simulink model "hcu_main_ADASwEPS"  (Simulink 8.2)
settings: Solver=FixedStepDiscrete  StartTime=0.0  StopTime=inf  FixedStep=0.001  RelTol=1e-3
PostLoadFcn:
  | , if any(exist('dsrtsu_mdlpostloadfcn', 'file') == [2, 3, 6]), try dsrtsu_mdlpostloadfcn('Execute', bdroot); catch fprintf('Error in PostLoadFcn (dsrtsu_mdlpostloadfcn) for model "%s":\n %s\n', bdroot, lasterr); end, end,
values from neighbouring files (symbols this model uses):
  C_TASK_1MS_S = (	C_TICK_TIME_S       )    [hcu_local_hdr.m]    (also in temp_ovrd_values.m = double(	0.001                  ))
  C_TASK_5MS_S = (	C_TICK_TIME_S      	)    [hcu_local_hdr.m]
  ENUM_ADASLFCSTATUS_OFF = uint8(  0  )    [hcu_local_hdr.m]
  ENUM_ADASLFCSTATUS_STANDBY = uint8(  1  )    [hcu_local_hdr.m]
  ENUM_ADASLKASTATUS_ACTIVE = uint8(  2  )    [hcu_local_hdr.m]
  ENUM_ADASLKASTATUS_OFF = uint8(  0  )    [hcu_local_hdr.m]
  ENUM_ADASLKASTATUS_STANDBY = uint8(  1  )    [hcu_local_hdr.m]
  ENUM_EPSMODEREQ_ANGLE = uint8(  1  )    [hcu_local_hdr.m]
  ENUM_EPSMODEREQ_INTERNAL = uint8(  0  )    [hcu_local_hdr.m]
  ENUM_EPSMODEREQ_TORQUE = uint8(  2  )    [hcu_local_hdr.m]
  ENUM_GEARPOSN_1ST = uint8(  1  )    [hcu_local_hdr.m]
  ENUM_GEARPOSN_2ND = uint8(  2  )    [hcu_local_hdr.m]
  ENUM_GEARPOSN_3RD = uint8(  3  )    [hcu_local_hdr.m]
  ENUM_GEARPOSN_4TH = uint8(  4  )    [hcu_local_hdr.m]
  ENUM_GEARPOSN_5TH = uint8(  5  )    [hcu_local_hdr.m]
  ENUM_GEARPOSN_6TH = uint8(  6  )    [hcu_local_hdr.m]
  ENUM_GEARPOSN_PN = uint8(  0  )    [hcu_local_hdr.m]
  ENUM_GEARPOSN_R = uint8(  7  )    [hcu_local_hdr.m]
  FALSE = boolean( 0 )    [hcu_local_hdr.m]
  TRUE = boolean( 1 )    [hcu_local_hdr.m]
undefined symbols (not defined in the file or in its folder): AACC_DistCtrlIMult_X_mps2, AACC_DistCtrlPMult_X_mps2, AACC_GearActual_enum, AACC_SpdCtrlIMult_X_mps2, AACC_SpdCtrlPMult_X_mps2, AACC_VehSpd_kph, AISP_EPSCurrent_pct, AISP_TqASensorDelta_pct, AISP_TqBSensorDelta_pct, ENUM_ACCSTATUS_ACTIVE, ENUM_ACCSTATUS_OFF, ENUM_ACCSTATUS_STANDBY, ENUM_ADASLFCSTATUS_ACTIVE, ENUM_ADASLFCSTATUS_TRANSITION, ENUM_LFCCCONTSTATUS_ACTIVE, ENUM_LFCCCONTSTATUS_NOTAVAIL_TEMP, ENUM_LFCCCONTSTATUS_OFF, ENUM_LFCCCONTSTATUS_READY, ENUM_LFCCCONTSTATUS_TRANSITION, ENUM_LKACCONTSTATUS_ACTIVE, ENUM_LKACCONTSTATUS_NOTAVAIL_TEMP, ENUM_LKACCONTSTATUS_OFF, ENUM_LKACCONTSTATUS_READY, KACC_AcclReqMax_g, KACC_AcclReqMin_g, KACC_ACCSetTimeGapDef1_s, KACC_ACCSetTimeGapDef2_s, KACC_ACCSetTimeGapDef3_s, KACC_ACCSetTimeGapDef4_s, KACC_ACCSetTimeGapDef5_s, KACC_AirDensity_kgpm3, KACC_AirDragCoef_rat, KACC_CommandsOn_flg, KACC_CruzSpdChgTimeThres_s, KACC_DecReqSwOffThres_Nm, KACC_DecReqSwOnThres_Nm, KACC_DistCtrlAdjTime_s, KACC_DistCtrlCalRate_s, KACC_DistCtrlIC_mps2, KACC_DistCtrlIGain_rat, KACC_DistCtrlIMax_mps2, KACC_DistCtrlIMin_mps2, KACC_DistCtrlIRest_flg, KACC_DistCtrlKGain_rat, KACC_DistCtrlPause_flg, KACC_DistCtrlPGain_rat, KACC_FinalDriveEff_pct, KACC_FinalDriveRatio_rat, KACC_FrontalArea_m2, KACC_GearBoxEff_pct, KACC_LongPushSpdChg_kph, KACC_MaxAccSetSpd_kph, KACC_MinAccSetSpd_kph, KACC_SetAllowSpdLim_kph, KACC_SpdCtrlAdjTime_s, KACC_SpdCtrlCalRate_s, KACC_SpdCtrlIC_mps2, KACC_SpdCtrlIGain_rat, KACC_SpdCtrlIMax_mps2, KACC_SpdCtrlIMin_mps2 ... (+26)
libraries: simulink x54, adas_lib x6, rti1401lib_dio_type3 x4, rtimmsu_dsrtlib x3, hcu_lib x2, aeb x1, ddm x1, dfr x1, dgi x1, dhp x1, dinr x1, dip x1
(part 6 of 9)

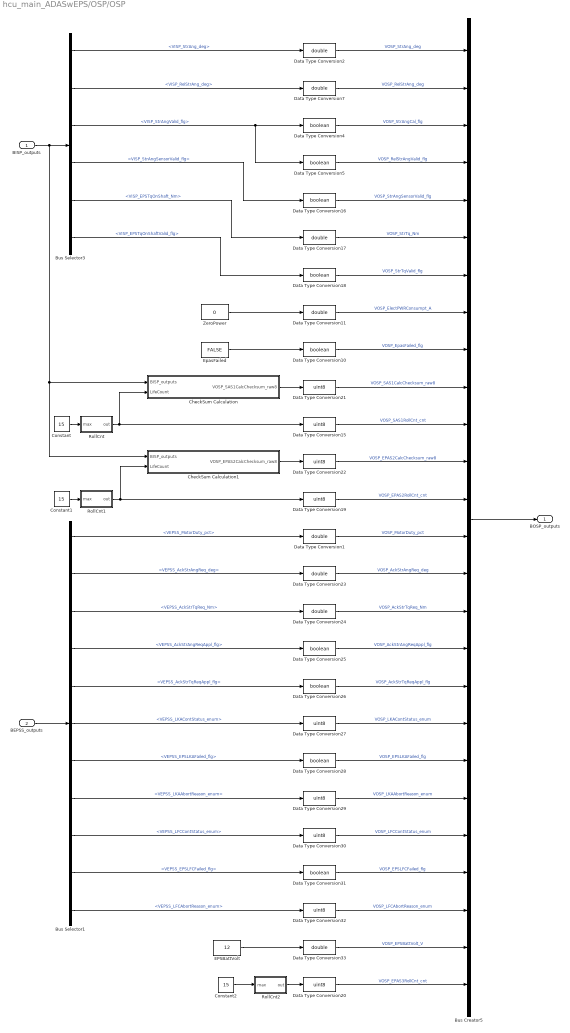
== system hcu_main_ADASwEPS/OSP/OSP ==
  BISP_outputs : Inport
  BEPSS_outputs : Inport  Port=2
  Bus Creator5 : BusCreator  Inputs=26
  Bus Selector1 : BusSelector  OutputSignals=VEPSS_MotorDuty_pct,VEPSS_AckStrAngReq_deg,VEPSS_AckStrTqReq_Nm,VEPSS_AckStrAngReqAppl_flg,VEPSS_AckStrTqReqAppl_flg,VEPSS_LKAContStatus_enum,VEPSS_EPSLKAFailed_flg,VEPSS_LKAAbortReason_enum,VEPSS_LFCContStatus_enum,VEPSS_EPSLFCFailed_flg,VEPSS_LFCAbortReason_enum
  Bus Selector3 : BusSelector  OutputSignals=VISP_StrAng_deg,VISP_RelStrAng_deg,VISP_StrAngValid_flg,VISP_StrAngSensorValid_flg,VISP_EPSTqOnShaft_Nm,VISP_EPSTqOnShaftValid_flg
  CheckSum Calculation : Subsystem  TreatAsAtomicUnit=on
  CheckSum Calculation1 : Subsystem  TreatAsAtomicUnit=on
  Constant : Constant  Value=15  OutDataTypeStr=uint8
  Constant1 : Constant  Value=15  OutDataTypeStr=uint8
  Constant2 : Constant  Value=15  OutDataTypeStr=uint8
  Data Type Conversion{1..2,7,11,17,23..24,33} (8 alike) : DataTypeConversion  OutDataTypeStr=double
  Data Type Conversion{4..5,10,16,18,25..26,28,31} (9 alike) : DataTypeConversion  OutDataTypeStr=boolean
  Data Type Conversion{15,19..22,27,29..30,32} (9 alike) : DataTypeConversion  OutDataTypeStr=uint8
  EPSBattVolt : Constant  Value=12
  EpasFailed : Constant  Value=FALSE
  RollCnt : Subsystem
  RollCnt1 : Subsystem
  RollCnt2 : Subsystem
  ZeroPower : Constant  Value=0
  BOSP_outputs : Outport
  wires:
  Bus Creator5/1 -> BOSP_outputs/1
  EpasFailed/1 -> Data Type Conversion10/1
  Data Type Conversion10/1 -> Bus Creator5/9  "VOSP_EpasFailed_flg"
  Data Type Conversion11/1 -> Bus Creator5/8  "VOSP_ElectPWRConsumpt_A"
  Data Type Conversion1/1 -> Bus Creator5/14  "VOSP_MotorDuty_pct"
  BEPSS_outputs/1 -> Bus Selector1/1
  Bus Selector1/1 -> Data Type Conversion1/1  "<VEPSS_MotorDuty_pct>"
  BISP_outputs/1 -> Bus Selector3/1, CheckSum Calculation/1(BISP_outputs), CheckSum Calculation1/1(BISP_outputs)
  Bus Selector3/1 -> Data Type Conversion2/1  "<VISP_StrAng_deg>"
  Data Type Conversion2/1 -> Bus Creator5/1  "VOSP_StrAng_deg"
  Bus Selector3/3 -> Data Type Conversion5/1, Data Type Conversion4/1  "<VISP_StrAngValid_flg>"
  Data Type Conversion4/1 -> Bus Creator5/3  "VOSP_StrAngCal_flg"
  Data Type Conversion5/1 -> Bus Creator5/4  "VOSP_RelStrAngValid_flg"
  Bus Selector3/2 -> Data Type Conversion7/1  "<VISP_RelStrAng_deg>"
  Data Type Conversion7/1 -> Bus Creator5/2  "VOSP_RelStrAng_deg"
  Bus Selector3/4 -> Data Type Conversion16/1  "<VISP_StrAngSensorValid_flg>"
  Data Type Conversion16/1 -> Bus Creator5/5  "VOSP_StrAngSensorValid_flg"
  Bus Selector3/5 -> Data Type Conversion17/1  "<VISP_EPSTqOnShaft_Nm>"
  Data Type Conversion17/1 -> Bus Creator5/6  "VOSP_StrTq_Nm"
  Bus Selector3/6 -> Data Type Conversion18/1  "<VISP_EPSTqOnShaftValid_flg>"
  Data Type Conversion18/1 -> Bus Creator5/7  "VOSP_StrTqValid_flg"
  ZeroPower/1 -> Data Type Conversion11/1
  Constant/1 -> RollCnt/1(max)
  RollCnt/1(out) -> Data Type Conversion15/1, CheckSum Calculation/2(LifeCount)
  Constant1/1 -> RollCnt1/1(max)
  RollCnt1/1(out) -> Data Type Conversion19/1, CheckSum Calculation1/2(LifeCount)
  Data Type Conversion15/1 -> Bus Creator5/11  "VOSP_SAS1RollCnt_cnt"
  Data Type Conversion19/1 -> Bus Creator5/13  "VOSP_EPAS2RollCnt_cnt"
  Constant2/1 -> RollCnt2/1(max)
  RollCnt2/1(out) -> Data Type Conversion20/1
  Data Type Conversion20/1 -> Bus Creator5/26  "VOSP_EPAS3RollCnt_cnt"
  CheckSum Calculation/1(VOSP_SAS1CalcChecksum_raw8) -> Data Type Conversion21/1
  Data Type Conversion21/1 -> Bus Creator5/10  "VOSP_SAS1CalcChecksum_raw8"
  Data Type Conversion22/1 -> Bus Creator5/12  "VOSP_EPAS2CalcChecksum_raw8"
  CheckSum Calculation1/1(VOSP_EPAS2CalcChecksum_raw8) -> Data Type Conversion22/1
  Bus Selector1/2 -> Data Type Conversion23/1  "<VEPSS_AckStrAngReq_deg>"
  Data Type Conversion23/1 -> Bus Creator5/15  "VOSP_AckStrAngReq_deg"
  Bus Selector1/3 -> Data Type Conversion24/1  "<VEPSS_AckStrTqReq_Nm>"
  Data Type Conversion24/1 -> Bus Creator5/16  "VOSP_AckStrTqReq_Nm"
  Bus Selector1/4 -> Data Type Conversion25/1  "<VEPSS_AckStrAngReqAppl_flg>"
  Data Type Conversion25/1 -> Bus Creator5/17  "VOSP_AckStrAngReqAppl_flg"
  Data Type Conversion26/1 -> Bus Creator5/18  "VOSP_AckStrTqReqAppl_flg"
  Bus Selector1/5 -> Data Type Conversion26/1  "<VEPSS_AckStrTqReqAppl_flg>"
  Bus Selector1/6 -> Data Type Conversion27/1  "<VEPSS_LKAContStatus_enum>"
  Data Type Conversion27/1 -> Bus Creator5/19  "VOSP_LKAContStatus_enum"
  Data Type Conversion28/1 -> Bus Creator5/20  "VOSP_EPSLKAFailed_flg"
  Bus Selector1/7 -> Data Type Conversion28/1  "<VEPSS_EPSLKAFailed_flg>"
  Data Type Conversion29/1 -> Bus Creator5/21  "VOSP_LKAAbortReason_enum"
  Bus Selector1/8 -> Data Type Conversion29/1  "<VEPSS_LKAAbortReason_enum>"
  Data Type Conversion30/1 -> Bus Creator5/22  "VOSP_LFCContStatus_enum"
  Data Type Conversion31/1 -> Bus Creator5/23  "VOSP_EPSLFCFailed_flg"
  Data Type Conversion32/1 -> Bus Creator5/24  "VOSP_LFCAbortReason_enum"
  Bus Selector1/9 -> Data Type Conversion30/1  "<VEPSS_LFCContStatus_enum>"
  Bus Selector1/10 -> Data Type Conversion31/1  "<VEPSS_EPSLFCFailed_flg>"
  Bus Selector1/11 -> Data Type Conversion32/1  "<VEPSS_LFCAbortReason_enum>"
  Data Type Conversion33/1 -> Bus Creator5/25  "VOSP_EPSBattVolt_V"
  EPSBattVolt/1 -> Data Type Conversion33/1

== system hcu_main_ADASwEPS/RTI Data/RTI Data Store ==
  RTI Data Store : Subsystem  mask(RTI_DATA_STORE){}
      mask help:
      | RTI Data Store Block. This block is used by RTI to store internal model dependent data. Deleting this block will result in data loss.
      |
      | NEVER DELETE, COPY, OR MODIFY THIS BLOCK!
      mask Help:
      | RTI Data Store Block. This block is used by RTI to store internal model dependent data. Deleting this block will result in data loss.
      | 
      | NEVER DELETE, COPY, OR MODIFY THIS BLOCK!
      mask Display: text(0.5, 0.5, ' ', 'HorizontalAlignment', 'center');

== system hcu_main_ADASwEPS/RTICANMM ControllerSetup/ModelClose ==

== system hcu_main_ADASwEPS/RTICANMM ControllerSetup1/ModelClose ==

== system hcu_main_ADASwEPS/RTICANMM GeneralSetup/ModelClose ==

== system hcu_main_ADASwEPS/User2CAN1__/ADAS1 ==
  BOUTP_outputs : Inport  OutDataTypeStr=Bus: BOUTP_outputs
  ADAS1_Checksum : Ground
  ADAS1_LifeCount : Ground
  ADAS_EPSMode : Ground
  ADAS_LFCMode : Ground
  ADAS_LFCStatus : Ground
  ADAS_LFCTransGain : Ground
  ADAS_LFCTransGain_A : Ground
  ADAS_LKAStatus : Ground
  Bus Selector : BusSelector  OutputSignals=VOUTP_StrTqAppl_flg,VOUTP_StrAngCmdValid_flg,VOUTP_StrTqReq_Nm,VOUTP_StrAngCmd_deg
  Data Type Conversion{,1..2,4} (4 alike) : DataTypeConversion
  buscreator : BusCreator  Inputs=12
  out : Outport
  wires:
  buscreator/1 -> out/1  "ADAS1"
  ADAS1_Checksum/1 -> buscreator/1  "ADAS1_Checksum"
  ADAS1_LifeCount/1 -> buscreator/2  "ADAS1_LifeCount"
  Data Type Conversion2/1 -> buscreator/3  "ADAS_StrTqReq_A"
  Data Type Conversion/1 -> buscreator/4  "ADAS_StrAngReq_A"
  ADAS_LFCTransGain_A/1 -> buscreator/5  "ADAS_LFCTransGain_A"
  ADAS_EPSMode/1 -> buscreator/6  "ADAS_EPSMode"
  ADAS_LKAStatus/1 -> buscreator/7  "ADAS_LKAStatus"
  ADAS_LFCMode/1 -> buscreator/8  "ADAS_LFCMode"
  ADAS_LFCStatus/1 -> buscreator/9  "ADAS_LFCStatus"
  Data Type Conversion4/1 -> buscreator/10  "ADAS_StrTqReq"
  ADAS_LFCTransGain/1 -> buscreator/11  "ADAS_LFCTransGain"
  Data Type Conversion1/1 -> buscreator/12  "ADAS_StrAngReq"
  BOUTP_outputs/1 -> Bus Selector/1
  Bus Selector/2 -> Data Type Conversion/1  "<VOUTP_StrAngCmdValid_flg>"
  Bus Selector/4 -> Data Type Conversion1/1  "<VOUTP_StrAngCmd_deg>"
  Bus Selector/1 -> Data Type Conversion2/1  "<VOUTP_StrTqAppl_flg>"
  Bus Selector/3 -> Data Type Conversion4/1  "<VOUTP_StrTqReq_Nm>"

== system hcu_main_ADASwEPS/User2CAN1__/ADAS2 ==
  BOUTP_outputs : Inport  OutDataTypeStr=Bus: BOUTP_outputs
  ADAS2_Checksum : Ground
  ADAS2_LifeCount : Ground
  Bus Selector : BusSelector  OutputSignals=VOUTP_VehHoldReq_flg,VOUTP_BrakePrefillReqAppl_flg,VOUTP_BrakePrefillReq_flg,VOUTP_AEBReqAppl_flg,VOUTP_AEBReq_flg,VOUTP_ForceIdleAppl_flg,VOUTP_DecReqProt_raw32,VOUTP_DecReq_mps2,VOUTP_DecReqAppl_flg,VOUTP_TqReqAppl_flg,VOUTP_ForceIdle_flg,VOUTP_TqReqProt_raw32,VOUTP_TqReq_Nm
  Data Type Conversion{,1..12} (13 alike) : DataTypeConversion
  buscreator : BusCreator  Inputs=15
  out : Outport
  wires:
  buscreator/1 -> out/1  "ADAS2"
  ADAS2_Checksum/1 -> buscreator/1  "ADAS2_Checksum"
  ADAS2_LifeCount/1 -> buscreator/2  "ADAS2_LifeCount"
  Data Type Conversion/1 -> buscreator/3  "ADAS_VehHoldReq"
  Data Type Conversion1/1 -> buscreator/4  "ADAS_BrakePrefillReq_A"
  Data Type Conversion2/1 -> buscreator/5  "ADAS_BrakePrefillReq"
  Data Type Conversion3/1 -> buscreator/6  "ADAS_AEBReq_A"
  Data Type Conversion4/1 -> buscreator/7  "ADAS_AEBReq"
  Data Type Conversion5/1 -> buscreator/8  "ADAS_ForceIdle_A"
  Data Type Conversion6/1 -> buscreator/9  "ADAS_DecReq_Prot"
  Data Type Conversion7/1 -> buscreator/10  "ADAS_DecReq"
  Data Type Conversion8/1 -> buscreator/11  "ADAS_DecReq_A"
  Data Type Conversion9/1 -> buscreator/12  "ADAS_TqReq_A"
  Data Type Conversion10/1 -> buscreator/13  "ADAS_ForceIdle"
  Data Type Conversion11/1 -> buscreator/14  "ADAS_TqReqProt"
  Data Type Conversion12/1 -> buscreator/15  "ADAS_TqReq"
  BOUTP_outputs/1 -> Bus Selector/1
  Bus Selector/4 -> Data Type Conversion3/1  "<VOUTP_AEBReqAppl_flg>"
  Bus Selector/3 -> Data Type Conversion2/1  "<VOUTP_BrakePrefillReq_flg>"
  Bus Selector/5 -> Data Type Conversion4/1  "<VOUTP_AEBReq_flg>"
  Bus Selector/6 -> Data Type Conversion5/1  "<VOUTP_ForceIdleAppl_flg>"
  Bus Selector/2 -> Data Type Conversion1/1  "<VOUTP_BrakePrefillReqAppl_flg>"
  Bus Selector/7 -> Data Type Conversion6/1  "<VOUTP_DecReqProt_raw32>"
  Bus Selector/1 -> Data Type Conversion/1  "<VOUTP_VehHoldReq_flg>"
  Bus Selector/8 -> Data Type Conversion7/1  "<VOUTP_DecReq_mps2>"
  Bus Selector/9 -> Data Type Conversion8/1  "<VOUTP_DecReqAppl_flg>"
  Bus Selector/10 -> Data Type Conversion9/1  "<VOUTP_TqReqAppl_flg>"
  Bus Selector/11 -> Data Type Conversion10/1  "<VOUTP_ForceIdle_flg>"
  Bus Selector/12 -> Data Type Conversion11/1  "<VOUTP_TqReqProt_raw32>"
  Bus Selector/13 -> Data Type Conversion12/1  "<VOUTP_TqReq_Nm>"

== system hcu_main_ADASwEPS/User2CAN1__/ADAS3 ==
  BOUTP_outputs : Inport  OutDataTypeStr=Bus: BOUTP_outputs
  ADAS3_Checksum : Ground
  ADAS3_LifeCount : Ground
  ADAS_GearPosnReq : Ground
  ADAS_GearPosnReq_A : Ground
  ADAS_MIL : Ground
  ADAS_ShftPosnReq : Ground
  ADAS_ShftPosnReq_A : Ground
  ADAS_VehSpdLim : Ground
  ADAS_VehSpdLim_A : Ground
  Bus Selector : BusSelector  OutputSignals=VOUTP_HazardWarningReq_flg
  Data Type Conversion : DataTypeConversion
  ForceLowBeam : Ground
  LeftTurnLightReq : Ground
  RightTurnLightReq : Ground
  buscreator : BusCreator  Inputs=13
  out : Outport
  wires:
  buscreator/1 -> out/1  "ADAS3"
  ADAS3_Checksum/1 -> buscreator/1  "ADAS3_Checksum"
  ADAS3_LifeCount/1 -> buscreator/2  "ADAS3_LifeCount"
  ForceLowBeam/1 -> buscreator/3  "ForceLowBeam"
  LeftTurnLightReq/1 -> buscreator/4  "LeftTurnLightReq"
  RightTurnLightReq/1 -> buscreator/5  "RightTurnLightReq"
  Data Type Conversion/1 -> buscreator/6  "HazardWarningReq"
  ADAS_MIL/1 -> buscreator/7  "ADAS_MIL"
  ADAS_ShftPosnReq_A/1 -> buscreator/8  "ADAS_ShftPosnReq_A"
  ADAS_ShftPosnReq/1 -> buscreator/9  "ADAS_ShftPosnReq"
  ADAS_VehSpdLim_A/1 -> buscreator/10  "ADAS_VehSpdLim_A"
  ADAS_GearPosnReq_A/1 -> buscreator/11  "ADAS_GearPosnReq_A"
  ADAS_GearPosnReq/1 -> buscreator/12  "ADAS_GearPosnReq"
  ADAS_VehSpdLim/1 -> buscreator/13  "ADAS_VehSpdLim"
  BOUTP_outputs/1 -> Bus Selector/1
  Bus Selector/1 -> Data Type Conversion/1  "<VOUTP_HazardWarningReq_flg>"

== system hcu_main_ADASwEPS/User2CAN1__/ADAS4 ==
  BOUTP_outputs : Inport  OutDataTypeStr=Bus: BOUTP_outputs
  ACCHMIWarningReq : Ground
  ADASFaultWarningReq : Ground
  AEBStatus : Ground
  APSEnable : Ground
  Bus Selector : BusSelector  OutputSignals=VOUTP_ACCStatus_enum,VOUTP_AEBWarningReq_flg,VOUTP_FCWWarningReq_flg
  Data Type Conversion : DataTypeConversion
  Data Type Conversion1 : DataTypeConversion
  Data Type Conversion2 : DataTypeConversion
  FCWStatus : Ground
  HapticWarningReq : Ground
  IGSAHMIWarningReq : Ground
  IGSAStatus : Ground
  LCSHMIWarningReq : Ground
  LCSStatus : Ground
  LFCHMIWarningReq : Ground
  LFCMode : Ground
  LFCStatus : Ground
  LKAHMIWarningReq : Ground
  LKAStatus : Ground
  MAPAHMIWarningReq : Ground
  MAPAStatus : Ground
  MAPPHMIWarningReq : Ground
  MAPPStatus : Ground
  PilotMode : Ground
  buscreator : BusCreator  Inputs=23
  out : Outport
  wires:
  buscreator/1 -> out/1  "ADAS4"
  ADASFaultWarningReq/1 -> buscreator/1  "ADASFaultWarningReq"
  HapticWarningReq/1 -> buscreator/2  "HapticWarningReq"
  APSEnable/1 -> buscreator/3  "APSEnable"
  PilotMode/1 -> buscreator/4  "PilotMode"
  IGSAStatus/1 -> buscreator/5  "IGSAStatus"
  LFCMode/1 -> buscreator/6  "LFCMode"
  MAPPStatus/1 -> buscreator/7  "MAPPStatus"
  MAPAStatus/1 -> buscreator/8  "MAPAStatus"
  LCSStatus/1 -> buscreator/9  "LCSStatus"
  LFCStatus/1 -> buscreator/10  "LFCStatus"
  LKAStatus/1 -> buscreator/11  "LKAStatus"
  Data Type Conversion/1 -> buscreator/12  "ACCStatus"
  FCWStatus/1 -> buscreator/13  "FCWStatus"
  AEBStatus/1 -> buscreator/14  "AEBStatus"
  MAPPHMIWarningReq/1 -> buscreator/15  "MAPPHMIWarningReq"
  MAPAHMIWarningReq/1 -> buscreator/16  "MAPAHMIWarningReq"
  LCSHMIWarningReq/1 -> buscreator/17  "LCSHMIWarningReq"
  LFCHMIWarningReq/1 -> buscreator/18  "LFCHMIWarningReq"
  LKAHMIWarningReq/1 -> buscreator/19  "LKAHMIWarningReq"
  IGSAHMIWarningReq/1 -> buscreator/20  "IGSAHMIWarningReq"
  Data Type Conversion1/1 -> buscreator/21  "AEBHMIWarningReq"
  ACCHMIWarningReq/1 -> buscreator/22  "ACCHMIWarningReq"
  Data Type Conversion2/1 -> buscreator/23  "FCWHMIWarningReq"
  BOUTP_outputs/1 -> Bus Selector/1
  Bus Selector/1 -> Data Type Conversion/1  "<VOUTP_ACCStatus_enum>"
  Bus Selector/2 -> Data Type Conversion1/1  "<VOUTP_AEBWarningReq_flg>"
  Bus Selector/3 -> Data Type Conversion2/1  "<VOUTP_FCWWarningReq_flg>"

== system hcu_main_ADASwEPS/User2CAN1__/ADAS5 ==
  BOUTP_outputs : Inport  OutDataTypeStr=Bus: BOUTP_outputs
  ADAS_FaultMode : Ground
  ADAS_LaneModeL : Ground
  ADAS_LaneModeR : Ground
  Bus Selector : BusSelector  OutputSignals=VOUTP_ACCSetTimeGapTmp_enum,VOUTP_ACCSetTimeGap_enum,VOUTP_ACCSetSpeed_kph
  Data Type Conversion : DataTypeConversion
  Data Type Conversion1 : DataTypeConversion
  Data Type Conversion2 : DataTypeConversion
  IGSASetSpeed : Ground
  LeadVehTimeGap : Ground
  SetVehTimeGap : Ground
  TargetType : Ground
  buscreator : BusCreator  Inputs=10
  out : Outport
  wires:
  buscreator/1 -> out/1  "ADAS5"
  ADAS_FaultMode/1 -> buscreator/1  "ADAS_FaultMode"
  ADAS_LaneModeR/1 -> buscreator/2  "ADAS_LaneModeR"
  ADAS_LaneModeL/1 -> buscreator/3  "ADAS_LaneModeL"
  Data Type Conversion/1 -> buscreator/4  "SeleTimeGapLvl"
  Data Type Conversion1/1 -> buscreator/5  "SetTimeGapLvl"
  IGSASetSpeed/1 -> buscreator/6  "IGSASetSpeed"
  Data Type Conversion2/1 -> buscreator/7  "ACCSetSpeed"
  SetVehTimeGap/1 -> buscreator/8  "SetVehTimeGap"
  LeadVehTimeGap/1 -> buscreator/9  "LeadVehTimeGap"
  TargetType/1 -> buscreator/10  "TargetType"
  BOUTP_outputs/1 -> Bus Selector/1
  Bus Selector/1 -> Data Type Conversion/1  "<VOUTP_ACCSetTimeGapTmp_enum>"
  Bus Selector/2 -> Data Type Conversion1/1  "<VOUTP_ACCSetTimeGap_enum>"
  Bus Selector/3 -> Data Type Conversion2/1  "<VOUTP_ACCSetSpeed_kph>"

== system hcu_main_ADASwEPS/User2CAN1__/EPAS2 ==
  BOSP_outputs : Inport
  Bus Selector : BusSelector  OutputSignals=VOSP_EPAS2CalcChecksum_raw8,VOSP_EPAS2RollCnt_cnt,VOSP_RelStrAng_deg,VOSP_StrTq_Nm,VOSP_StrTqValid_flg,VOSP_RelStrAngValid_flg,VOSP_EpasFailed_flg,VOSP_ElectPWRConsumpt_A
  Logical Operator : Logic  Operator=NOT  AllPortsSameDT=off  OutDataTypeStr=boolean
  buscreator : BusCreator  Inputs=8
  dt_Elect_PWR_Consumpt : DataTypeConversion  RndMeth=Zero
  dt_EpasFailed : DataTypeConversion  RndMeth=Zero
  dt_RSP_OK : DataTypeConversion  RndMeth=Zero
  dt_R_SAS_Angle : DataTypeConversion  RndMeth=Zero
  dt_SAS_CheckSum2 : DataTypeConversion  RndMeth=Zero
  dt_SAS_MsgCount2 : DataTypeConversion  RndMeth=Zero
  dt_Steering_Torque : DataTypeConversion  RndMeth=Zero
  dt_Steering_Torque_V : DataTypeConversion  RndMeth=Zero
  out : Outport
  wires:
  buscreator/1 -> out/1  "EPAS2"
  dt_SAS_CheckSum2/1 -> buscreator/1  "SAS_CheckSum2"
  dt_SAS_MsgCount2/1 -> buscreator/2  "SAS_MsgCount2"
  dt_R_SAS_Angle/1 -> buscreator/3  "R_SAS_Angle"
  dt_Steering_Torque/1 -> buscreator/4  "Steering_Torque"
  dt_Steering_Torque_V/1 -> buscreator/5  "Steering_Torque_V"
  dt_RSP_OK/1 -> buscreator/6  "RSP_OK"
  dt_EpasFailed/1 -> buscreator/7  "EpasFailed"
  dt_Elect_PWR_Consumpt/1 -> buscreator/8  "Elect_PWR_Consumpt"
  Bus Selector/1 -> dt_SAS_CheckSum2/1  "<VOSP_EPAS2CalcChecksum_raw8>"
  Bus Selector/2 -> dt_SAS_MsgCount2/1  "<VOSP_EPAS2RollCnt_cnt>"
  Bus Selector/3 -> dt_R_SAS_Angle/1  "<VOSP_RelStrAng_deg>"
  Bus Selector/4 -> dt_Steering_Torque/1  "<VOSP_StrTq_Nm>"
  Bus Selector/5 -> Logical Operator/1  "<VOSP_StrTqValid_flg>"
  Bus Selector/6 -> dt_RSP_OK/1  "<VOSP_RelStrAngValid_flg>"
  Bus Selector/7 -> dt_EpasFailed/1  "<VOSP_EpasFailed_flg>"
  Bus Selector/8 -> dt_Elect_PWR_Consumpt/1  "<VOSP_ElectPWRConsumpt_A>"
  BOSP_outputs/1 -> Bus Selector/1
  Logical Operator/1 -> dt_Steering_Torque_V/1

== system hcu_main_ADASwEPS/User2CAN1__/EPAS3 ==
  BOSP_outputs : Inport
  Bus Selector : BusSelector  OutputSignals=VOSP_EPAS3RollCnt_cnt,VOSP_EPSLFCFailed_flg,VOSP_AckStrTqReqAppl_flg,VOSP_AckStrAngReqAppl_flg,VOSP_LFCContStatus_enum,VOSP_EPSBattVolt_V,VOSP_AckStrTqReq_Nm,VOSP_LFCAbortReason_enum,VOSP_LKAAbortReason_enum,VOSP_EPSLKAFailed_flg,VOSP_LKAContStatus_enum,VOSP_AckStrAngReq_deg
  Constant : Constant  Value=0
  Constant1 : Constant  Value=0
  Constant2 : Constant  Value=0
  buscreator : BusCreator  Inputs=15
  dt_SAS_CheckSum{1..15} (15 alike) : DataTypeConversion  RndMeth=Zero
  out : Outport
  wires:
  buscreator/1 -> out/1  "EPAS3"
  dt_SAS_CheckSum2/1 -> buscreator/1  "EPAS3_Checksum"
  dt_SAS_CheckSum1/1 -> buscreator/2  "EPAS3_LifeCount"
  dt_SAS_CheckSum3/1 -> buscreator/3  "EPSLFCFailed"
  dt_SAS_CheckSum4/1 -> buscreator/4  "CurStrTqReq_A"
  dt_SAS_CheckSum5/1 -> buscreator/5  "CurStrAngReq_A"
  dt_SAS_CheckSum6/1 -> buscreator/6  "EPSLFCStatus"
  dt_SAS_CheckSum7/1 -> buscreator/7  "EPSBattVolt"
  dt_SAS_CheckSum8/1 -> buscreator/8  "CurStrTqReq"
  dt_SAS_CheckSum9/1 -> buscreator/9  "DriverStrIntdLvl"
  dt_SAS_CheckSum10/1 -> buscreator/10  "DriverStrIntd"
  dt_SAS_CheckSum11/1 -> buscreator/11  "EPSLFCAbReason"
  dt_SAS_CheckSum12/1 -> buscreator/12  "EPSLKAAbReason"
  dt_SAS_CheckSum13/1 -> buscreator/13  "EPSLKAFailed"
  dt_SAS_CheckSum14/1 -> buscreator/14  "EPSLKAStatus"
  dt_SAS_CheckSum15/1 -> buscreator/15  "CurStrAngReq"
  BOSP_outputs/1 -> Bus Selector/1
  Bus Selector/1 -> dt_SAS_CheckSum1/1  "<VOSP_EPAS3RollCnt_cnt>"
  Constant/1 -> dt_SAS_CheckSum2/1
  Bus Selector/2 -> dt_SAS_CheckSum3/1  "<VOSP_EPSLFCFailed_flg>"
  Bus Selector/3 -> dt_SAS_CheckSum4/1  "<VOSP_AckStrTqReqAppl_flg>"
  Bus Selector/4 -> dt_SAS_CheckSum5/1  "<VOSP_AckStrAngReqAppl_flg>"
  Bus Selector/5 -> dt_SAS_CheckSum6/1  "<VOSP_LFCContStatus_enum>"
  Bus Selector/6 -> dt_SAS_CheckSum7/1  "<VOSP_EPSBattVolt_V>"
  Bus Selector/7 -> dt_SAS_CheckSum8/1  "<VOSP_AckStrTqReq_Nm>"
  Bus Selector/8 -> dt_SAS_CheckSum11/1  "<VOSP_LFCAbortReason_enum>"
  Bus Selector/9 -> dt_SAS_CheckSum12/1  "<VOSP_LKAAbortReason_enum>"
  Bus Selector/10 -> dt_SAS_CheckSum13/1  "<VOSP_EPSLKAFailed_flg>"
  Bus Selector/11 -> dt_SAS_CheckSum14/1  "<VOSP_LKAContStatus_enum>"
  Bus Selector/12 -> dt_SAS_CheckSum15/1  "<VOSP_AckStrAngReq_deg>"
  Constant1/1 -> dt_SAS_CheckSum9/1
  Constant2/1 -> dt_SAS_CheckSum10/1

== system hcu_main_ADASwEPS/User2CAN1__/SAS1 ==
  BOSP_outputs : Inport
  Bus Selector : BusSelector  OutputSignals=VOSP_SAS1CalcChecksum_raw8,VOSP_SAS1RollCnt_cnt,VOSP_StrAngSensorValid_flg,VOSP_StrAngCal_flg,VOSP_StrAng_deg
  buscreator : BusCreator  Inputs=5
  dt_SAS_Angle : DataTypeConversion  RndMeth=Zero
  dt_SAS_CAL : DataTypeConversion  RndMeth=Zero
  dt_SAS_CheckSum : DataTypeConversion  RndMeth=Zero
  dt_SAS_MsgCount : DataTypeConversion  RndMeth=Zero
  dt_SAS_OK : DataTypeConversion  RndMeth=Zero
  out : Outport
  wires:
  buscreator/1 -> out/1  "SAS1"
  dt_SAS_CheckSum/1 -> buscreator/1  "SAS_CheckSum"
  dt_SAS_MsgCount/1 -> buscreator/2  "SAS_MsgCount"
  dt_SAS_OK/1 -> buscreator/3  "SAS_OK"
  dt_SAS_CAL/1 -> buscreator/4  "SAS_CAL"
  dt_SAS_Angle/1 -> buscreator/5  "SAS_Angle"
  Bus Selector/3 -> dt_SAS_OK/1  "<VOSP_StrAngSensorValid_flg>"
  Bus Selector/2 -> dt_SAS_MsgCount/1  "<VOSP_SAS1RollCnt_cnt>"
  Bus Selector/4 -> dt_SAS_CAL/1  "<VOSP_StrAngCal_flg>"
  Bus Selector/1 -> dt_SAS_CheckSum/1  "<VOSP_SAS1CalcChecksum_raw8>"
  Bus Selector/5 -> dt_SAS_Angle/1  "<VOSP_StrAng_deg>"
  BOSP_outputs/1 -> Bus Selector/1

== system hcu_main_ADASwEPS/User2RTICANMM MainBlock_/ABS2_C ==
  CAN1_Rx1 : Inport
  Bus Selector2 : BusSelector  OutputSignals=ABS2.BrkSw_Sta,ABS2.BrkSw_V,ABS2.VehSpeed
  Data Type Conversion3 : DataTypeConversion
  Data Type Conversion4 : DataTypeConversion
  Data Type Conversion5 : DataTypeConversion
  buscreator : BusCreator  Inputs=3
  out : Outport
  wires:
  buscreator/1 -> out/1  "ABS2_C"
  Data Type Conversion3/1 -> buscreator/1  "BrkSw_Sta"
  Data Type Conversion4/1 -> buscreator/2  "BrkSw_V"
  Data Type Conversion5/1 -> buscreator/3  "VehSpeed"
  Bus Selector2/1 -> Data Type Conversion3/1  "<BrkSw_Sta>"
  Bus Selector2/2 -> Data Type Conversion4/1  "<BrkSw_V>"
  Bus Selector2/3 -> Data Type Conversion5/1  "<VehSpeed>"
  CAN1_Rx1/1 -> Bus Selector2/1

== system hcu_main_ADASwEPS/User2RTICANMM MainBlock_/ABS4_C ==
  CAN1_Rx : Inport
  Bus Selector1 : BusSelector  OutputSignals=ABS4.YawRate,SAS1.SAS_Angle,SAS1.SAS_OK,ABS4.YawRate_V,SAS1.SAS_CAL
  Data Type Conversion{,1..4} (5 alike) : DataTypeConversion
  Logical Operator : Logic  Operator=NOT  AllPortsSameDT=off  OutDataTypeStr=boolean
  Logical Operator1 : Logic  Operator=NOT  AllPortsSameDT=off  OutDataTypeStr=boolean
  buscreator : BusCreator  Inputs=5
  out : Outport
  wires:
  buscreator/1 -> out/1  "ABS4_C"
  Data Type Conversion/1 -> buscreator/1  "YawRate"
  Data Type Conversion1/1 -> buscreator/2  "SteerAng"
  Data Type Conversion2/1 -> buscreator/3  "SteerAng_Sensor_V"
  Data Type Conversion3/1 -> buscreator/4  "YawRate_V"
  Data Type Conversion4/1 -> buscreator/5  "SteerAng_V"
  CAN1_Rx/1 -> Bus Selector1/1
  Logical Operator/1 -> Data Type Conversion2/1
  Bus Selector1/1 -> Data Type Conversion/1  "<YawRate>"
  Bus Selector1/2 -> Data Type Conversion1/1  "<SAS_Angle>"
  Bus Selector1/3 -> Logical Operator/1  "<SAS_OK>"
  Bus Selector1/4 -> Data Type Conversion3/1  "<YawRate_V>"
  Bus Selector1/5 -> Logical Operator1/1  "<SAS_CAL>"
  Logical Operator1/1 -> Data Type Conversion4/1

== system hcu_main_ADASwEPS/User2RTICANMM MainBlock_/SAS1_C ==
  CAN1_Rx : Inport
  Bus Selector1 : BusSelector  OutputSignals=SAS1.SAS_CheckSum,SAS1.SAS_MsgCount,SAS1.SAS_OK,SAS1.SAS_CAL,SAS1.SAS_Angle
  Data Type Conversion{1..5} (5 alike) : DataTypeConversion
  buscreator : BusCreator  Inputs=5
  out : Outport
  wires:
  buscreator/1 -> out/1  "SAS1"
  Data Type Conversion1/1 -> buscreator/1  "SAS_CheckSum"
  Data Type Conversion2/1 -> buscreator/2  "SAS_MsgCount"
  Data Type Conversion3/1 -> buscreator/3  "SAS_OK"
  Data Type Conversion4/1 -> buscreator/4  "SAS_CAL"
  Data Type Conversion5/1 -> buscreator/5  "SAS_Angle"
  CAN1_Rx/1 -> Bus Selector1/1
  Bus Selector1/1 -> Data Type Conversion1/1  "<SAS_CheckSum>"
  Bus Selector1/2 -> Data Type Conversion2/1  "<SAS_MsgCount>"
  Bus Selector1/3 -> Data Type Conversion3/1  "<SAS_OK>"
  Bus Selector1/4 -> Data Type Conversion4/1  "<SAS_CAL>"
  Bus Selector1/5 -> Data Type Conversion5/1  "<SAS_Angle>"

== system hcu_main_ADASwEPS/User2RTICANMM MainBlock_/SpeedInformation ==
  CAN1_Rx : Inport
  Bus Selector1 : BusSelector  OutputSignals=ABS2.VehSpeed
  Bus Selector2 : BusSelector  OutputSignals=TCM1.CAN_GEAR_STATE_NOW
  Constant : Constant  Value=single(0)
  Constant1 : Constant  Value=uint8(0)
  Constant10 : Constant  Value=uint8(2)
  Constant11 : Constant  Value=uint8(3)
  Constant2 : Constant  Value=ENUM_GEARPOSN_1ST
  Constant3 : Constant  Value=ENUM_GEARPOSN_2ND
  Constant4 : Constant  Value=ENUM_GEARPOSN_3RD
  Constant5 : Constant  Value=ENUM_GEARPOSN_4TH
  Constant6 : Constant  Value=ENUM_GEARPOSN_5TH
  Constant7 : Constant  Value=ENUM_GEARPOSN_6TH
  Constant8 : Constant  Value=ENUM_GEARPOSN_R
  Constant9 : Constant  Value=uint8(1)
  Data Type Conversion1 : DataTypeConversion
  Data Type Conversion2 : DataTypeConversion
  Gain : Gain  Gain=1000/3600
  Logical Operator : Logic  Operator=OR  Inputs=6  AllPortsSameDT=off  OutDataTypeStr=boolean
  Relational Operator{,1..7} (8 alike) : RelationalOperator  Operator===  OutDataTypeStr=boolean
  Switch : Switch  Criteria=u2 ~= 0
  Switch1 : Switch  Criteria=u2 ~= 0
  Switch2 : Switch  Criteria=u2 ~= 0
  buscreator : BusCreator  Inputs=2
  out : Outport
  wires:
  buscreator/1 -> out/1  "SpeedInformation"
  Data Type Conversion2/1 -> buscreator/2  "radarDeviceSpeedDirection"
  Data Type Conversion1/1 -> buscreator/1  "radarDeviceSpeed"
  CAN1_Rx/1 -> Bus Selector2/1, Bus Selector1/1
  Bus Selector1/1 -> Relational Operator/1, Gain/1  "<VehSpeed>"
  Bus Selector2/1 -> Relational Operator3/1, Relational Operator4/1, Relational Operator5/1, Relational Operator6/1, Relational Operator7/1, Relational Operator2/1, Relational Operator1/1  "<CAN_GEAR_STATE_NOW>"
  Gain/1 -> Data Type Conversion1/1
  Switch/1 -> Data Type Conversion2/1
  Relational Operator/1 -> Switch/2
  Constant/1 -> Relational Operator/2
  Constant1/1 -> Switch/1
  Constant2/1 -> Relational Operator1/2
  Constant3/1 -> Relational Operator2/2
  Constant4/1 -> Relational Operator3/2
  Constant5/1 -> Relational Operator4/2
  Constant6/1 -> Relational Operator5/2
  Constant7/1 -> Relational Operator6/2
  Constant8/1 -> Relational Operator7/2
  Relational Operator1/1 -> Logical Operator/1
  Relational Operator2/1 -> Logical Operator/2
  Relational Operator3/1 -> Logical Operator/3
  Relational Operator4/1 -> Logical Operator/4
  Relational Operator5/1 -> Logical Operator/5
  Relational Operator6/1 -> Logical Operator/6
  Switch1/1 -> Switch/3
  Logical Operator/1 -> Switch1/2
  Constant9/1 -> Switch1/1
  Switch2/1 -> Switch1/3
  Relational Operator7/1 -> Switch2/2
  Constant10/1 -> Switch2/1
  Constant11/1 -> Switch2/3

== system hcu_main_ADASwEPS/User2RTICANMM MainBlock_/YawRateInformation ==
  CAN1_Rx : Inport
  Bus Selector1 : BusSelector  OutputSignals=ABS4.YawRate
  Data Type Conversion1 : DataTypeConversion
  Gain : Gain  Gain=-1
  buscreator : BusCreator  Inputs=1
  out : Outport
  wires:
  buscreator/1 -> out/1  "YawRateInformation"
  Data Type Conversion1/1 -> buscreator/1  "radarDeviceYawRate"
  CAN1_Rx/1 -> Bus Selector1/1
  Bus Selector1/1 -> Gain/1  "<YawRate>"
  Gain/1 -> Data Type Conversion1/1

== system hcu_main_ADASwEPS/APPH/ACC/ACC ==
  VDINR_DriverBrakPedalOn_flg : Inport
  VDINR_VehSpd_kph : Inport  Port=2
  VDINR_ACCOnVCU_flg : Inport  Port=3
  VDINR_ACCResSpdIncVCU_flg : Inport  Port=4
  VDINR_ACCSetSpdDecVCU_flg : Inport  Port=5
  VDINR_ACCTimeGapIncVCU_flg : Inport  Port=6
  VDINR_ACCTimeGapDecVCU_flg : Inport  Port=7
  VDINR_NowGearPosn_enum : Inport  Port=8
  VDINR_EngSpd_rpm : Inport  Port=9
  VDINR_DefMaxACCSetSpeed_kph : Inport  Port=10
  VMCT_MCTPositionX_m : Inport  Port=11
  VMCT_MCTRelVelocityX_mps : Inport  Port=12
  VMCT_MCTInPath_flg : Inport  Port=13
  VAEB_AEBActive_flg : Inport  Port=14
  ACCStatus_SetSpeed_SetTimeGap : Subsystem  TreatAsAtomicUnit=on
  ACCStrategy : Subsystem
  CommandDetermination : Subsystem
  VACC_ACCStatus_enum : Outport
  VACC_ACCSetTimeGap_enum : Outport  Port=2
  VACC_ACCSetTimeGapTmp_enum : Outport  Port=3
  VACC_ACCSetSpd_kph : Outport  Port=4
  VACC_TqReq_Nm : Outport  Port=5
  VACC_TqReqAppl_flg : Outport  Port=6
  VACC_DecReq_mps2 : Outport  Port=7
  VACC_DecReqAppl_flg : Outport  Port=8
  wires:
  VDINR_DriverBrakPedalOn_flg/1 -> ACCStatus_SetSpeed_SetTimeGap/1(VDINR_DriverBrakPedalOn_flg)
  VDINR_VehSpd_kph/1 -> [VDINR_VehSpd_kph], ACCStatus_SetSpeed_SetTimeGap/3(VDINR_VehSpd_kph)
  VDINR_ACCOnVCU_flg/1 -> ACCStatus_SetSpeed_SetTimeGap/4(VDINR_ACCOnVCU_flg)
  VDINR_ACCResSpdIncVCU_flg/1 -> ACCStatus_SetSpeed_SetTimeGap/5(VDINR_ACCResSpdIncVCU_flg)
  VDINR_ACCSetSpdDecVCU_flg/1 -> ACCStatus_SetSpeed_SetTimeGap/6(VDINR_ACCSetSpdDecVCU_flg)
  VDINR_ACCTimeGapIncVCU_flg/1 -> ACCStatus_SetSpeed_SetTimeGap/7(VDINR_ACCTimeGapIncVCU_flg)
  VDINR_ACCTimeGapDecVCU_flg/1 -> ACCStatus_SetSpeed_SetTimeGap/8(VDINR_ACCTimeGapDecVCU_flg)
  ACCStatus_SetSpeed_SetTimeGap/1(VACC_ACCStatus_enum) -> VACC_ACCStatus_enum/1
  ACCStatus_SetSpeed_SetTimeGap/5(VACC_ACCSetSpd_kph) -> [VACC_ACCSetSpd_kph], ACCStrategy/1(VACC_ACCSetSpd_kph)
  ACCStatus_SetSpeed_SetTimeGap/6(VACC_ACCSetTimeGap_s) -> ACCStrategy/2(VACC_ACCSetTimeGap_s)
  ACCStatus_SetSpeed_SetTimeGap/4(VACC_ACCActivated_flg) -> CommandDetermination/1(VACC_ACCActivated_flg), ACCStrategy/Enable
  [VDINR_VehSpd_kph] -> ACCStrategy/3(VDINR_VehSpd_kph)
  VMCT_MCTPositionX_m/1 -> ACCStrategy/4(VMCT_MCTPositionX_m)
  VMCT_MCTRelVelocityX_mps/1 -> ACCStrategy/5(VMCT_MCTRelVelocityX_mps)
  VDINR_NowGearPosn_enum/1 -> [VDINR_NowGearPosn_enum], ACCStrategy/6(VDINR_NowGearPosn_enum)
  VDINR_EngSpd_rpm/1 -> ACCStrategy/7(VDINR_EngSpd_rpm)
  ACCStrategy/1(VACC_TqReqRaw_Nm) -> CommandDetermination/2(VACC_TqReqRaw_Nm)
  ACCStrategy/2(VACC_AcclReqFinal_mps2) -> CommandDetermination/3(VACC_AcclReq_mps2)
  CommandDetermination/1(VACC_TqReq_Nm) -> VACC_TqReq_Nm/1
  CommandDetermination/4(VACC_DecReqAppl_flg) -> VACC_DecReqAppl_flg/1
  CommandDetermination/2(VACC_TqReqAppl_flg) -> VACC_TqReqAppl_flg/1
  CommandDetermination/3(VACC_DecReq_mps2) -> VACC_DecReq_mps2/1
  VMCT_MCTInPath_flg/1 -> ACCStrategy/8(VMCT_MCTInPath_flg)
  VDINR_DefMaxACCSetSpeed_kph/1 -> ACCStatus_SetSpeed_SetTimeGap/9(VDINR_DefMaxACCSetSpeed_kph)
  ACCStatus_SetSpeed_SetTimeGap/2(VACC_ACCSetTimeGap_enum) -> VACC_ACCSetTimeGap_enum/1
  ACCStatus_SetSpeed_SetTimeGap/3(VACC_ACCSetTimeGapTmp_enum) -> VACC_ACCSetTimeGapTmp_enum/1
  [VACC_ACCSetSpd_kph] -> VACC_ACCSetSpd_kph/1
  [VDINR_NowGearPosn_enum] -> ACCStatus_SetSpeed_SetTimeGap/10(VDINR_NowGearPosn_enum)
  VAEB_AEBActive_flg/1 -> ACCStatus_SetSpeed_SetTimeGap/2(VAEB_AEBActive_flg)

== system hcu_main_ADASwEPS/APPH/ACC/model_info ==
  EmptySubsystem : Subsystem

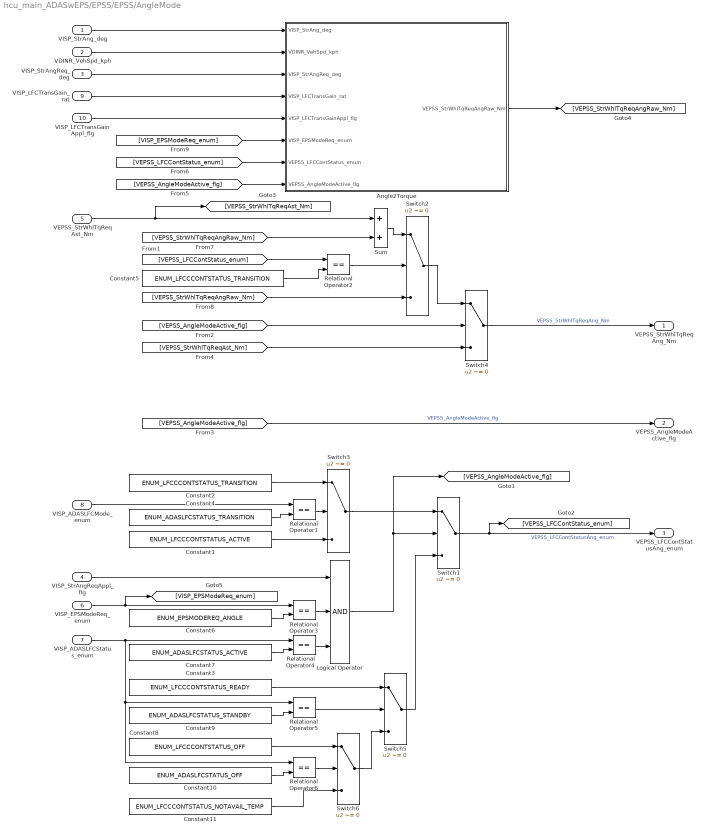
== system hcu_main_ADASwEPS/EPSS/EPSS/AngleMode ==
  VISP_StrAng_deg : Inport
  VDINR_VehSpd_kph : Inport  Port=2
  VISP_StrAngReq_deg : Inport  Port=3
  VISP_StrAngReqAppl_flg : Inport  Port=4
  VEPSS_StrWhlTqReqAst_Nm : Inport  Port=5
  VISP_EPSModeReq_enum : Inport  Port=6
  VISP_ADASLFCStatus_enum : Inport  Port=7
  VISP_ADASLFCMode_enum : Inport  Port=8
  VISP_LFCTransGain_rat : Inport  Port=9
  VISP_LFCTransGainAppl_flg : Inport  Port=10
  Angle2Torque : Subsystem
  Constant1 : Constant  Value=ENUM_LFCCCONTSTATUS_ACTIVE
  Constant10 : Constant  Value=ENUM_ADASLFCSTATUS_OFF
  Constant11 : Constant  Value=ENUM_LFCCCONTSTATUS_NOTAVAIL_TEMP
  Constant2 : Constant  Value=ENUM_LFCCCONTSTATUS_TRANSITION
  Constant3 : Constant  Value=ENUM_LFCCCONTSTATUS_READY
  Constant4 : Constant  Value=ENUM_ADASLFCSTATUS_TRANSITION
  Constant5 : Constant  Value=ENUM_LFCCCONTSTATUS_TRANSITION
  Constant6 : Constant  Value=ENUM_EPSMODEREQ_ANGLE
  Constant7 : Constant  Value=ENUM_ADASLFCSTATUS_ACTIVE
  Constant8 : Constant  Value=ENUM_LFCCCONTSTATUS_OFF
  Constant9 : Constant  Value=ENUM_ADASLFCSTATUS_STANDBY
  Logical Operator : Logic  Inputs=3  AllPortsSameDT=off  OutDataTypeStr=boolean
  Relational Operator{1..6} (6 alike) : RelationalOperator  Operator===  OutDataTypeStr=boolean
  Sum : Sum
  Switch{1..6} (6 alike) : Switch  Criteria=u2 ~= 0
  VEPSS_StrWhlTqReqAng_Nm : Outport
  VEPSS_AngleModeActive_flg : Outport  Port=2
  VEPSS_LFCContStatusAng_enum : Outport  Port=3
  wires:
  Constant11/1 -> Switch6/3
  Constant8/1 -> Switch6/1
  Relational Operator6/1 -> Switch6/2
  Constant10/1 -> Relational Operator6/2
  VISP_ADASLFCStatus_enum/1 -> Relational Operator4/1, Relational Operator5/1, Relational Operator6/1
  Switch6/1 -> Switch5/3
  Constant3/1 -> Switch5/1
  Relational Operator5/1 -> Switch5/2
  Constant9/1 -> Relational Operator5/2
  Switch5/1 -> Switch1/3
  Relational Operator4/1 -> Logical Operator/3
  Constant7/1 -> Relational Operator4/2
  Relational Operator3/1 -> Logical Operator/2
  Logical Operator/1 -> [VEPSS_AngleModeActive_flg], Switch1/2
  VISP_StrAngReqAppl_flg/1 -> Logical Operator/1
  Constant6/1 -> Relational Operator3/2
  VISP_EPSModeReq_enum/1 -> [VISP_EPSModeReq_enum], Relational Operator3/1
  [VEPSS_AngleModeActive_flg] -> VEPSS_AngleModeActive_flg/1  "VEPSS_AngleModeActive_flg"
  [VEPSS_StrWhlTqReqAst_Nm] -> Switch4/3
  Relational Operator2/1 -> Switch2/2
  [VEPSS_LFCContStatus_enum] -> Relational Operator2/1
  [VEPSS_AngleModeActive_flg] -> Switch4/2
  Constant2/1 -> Switch3/1
  Relational Operator1/1 -> Switch3/2
  Switch3/1 -> Switch1/1
  Constant4/1 -> Relational Operator1/2
  VISP_ADASLFCMode_enum/1 -> Relational Operator1/1
  Switch2/1 -> Switch4/1
  VEPSS_StrWhlTqReqAst_Nm/1 -> Sum/1, [VEPSS_StrWhlTqReqAst_Nm]
  Switch1/1 -> [VEPSS_LFCContStatus_enum], VEPSS_LFCContStatusAng_enum/1  "VEPSS_LFCContStatusAng_enum"
  Constant1/1 -> Switch3/3
  Switch4/1 -> VEPSS_StrWhlTqReqAng_Nm/1  "VEPSS_StrWhlTqReqAng_Nm"
  Sum/1 -> Switch2/1
  Constant5/1 -> Relational Operator2/2
  VISP_StrAngReq_deg/1 -> Angle2Torque/3(VISP_StrAngReq_deg)
  VISP_StrAng_deg/1 -> Angle2Torque/1(VISP_StrAng_deg)
  VDINR_VehSpd_kph/1 -> Angle2Torque/2(VDINR_VehSpd_kph)
  [VEPSS_AngleModeActive_flg] -> Angle2Torque/8(VEPSS_AngleModeActive_flg)
  Angle2Torque/1(VEPSS_StrWhlTqReqAngRaw_Nm) -> [VEPSS_StrWhlTqReqAngRaw_Nm]
  [VEPSS_LFCContStatus_enum] -> Angle2Torque/7(VEPSS_LFCContStatus_enum)
  [VEPSS_StrWhlTqReqAngRaw_Nm] -> Sum/2
  [VEPSS_StrWhlTqReqAngRaw_Nm] -> Switch2/3
  VISP_LFCTransGain_rat/1 -> Angle2Torque/4(VISP_LFCTransGain_rat)
  VISP_LFCTransGainAppl_flg/1 -> Angle2Torque/5(VISP_LFCTransGainAppl_flg)
  [VISP_EPSModeReq_enum] -> Angle2Torque/6(VISP_EPSModeReq_enum)

== system hcu_main_ADASwEPS/EPSS/EPSS/EPSMotorPWMRequest ==
  VEPSS_StrWhlTqReqAst_Nm : Inport
  VEPSS_StrWhlTqReqTq_Nm : Inport  Port=2
  VEPSS_StrWhlTqReqAng_Nm : Inport  Port=3
  VEPSS_LFCContStatus_enum : Inport  Port=4
  VEPSS_TorqueModeActive_flg : Inport  Port=5
  VEPSS_AngleModeActive_flg : Inport  Port=6
  VISP_VehSpd_kph : Inport  Port=7
  VISP_LFCTransGain_rat : Inport  Port=8
  VISP_LFCTransGainAppl_flg : Inport  Port=9
  VISP_EPSModeReq_enum : Inport  Port=10
  VISP_EPSTqOnShaftValid_flg : Inport  Port=11
  EPSControl_Off : Constant  Value=0
  MotorPWMRequestCalculation : Subsystem
  MotorTorqueRequestCalculation : Subsystem
  Switch2 : Switch  Criteria=u2 ~= 0
  VEPSS_EPSMotPWMReq_pct : Outport
  wires:
  EPSControl_Off/1 -> Switch2/3
  VEPSS_LFCContStatus_enum/1 -> MotorTorqueRequestCalculation/9(VEPSS_LFCContStatus_enum)
  Switch2/1 -> VEPSS_EPSMotPWMReq_pct/1  "VEPSS_EPSMotPWMReq_pct"
  MotorTorqueRequestCalculation/1(VEPSS_EPSMotTqReq_Nm) -> MotorPWMRequestCalculation/1(VEPSS_EPSMotTqReqRaw_Nm)
  VISP_EPSTqOnShaftValid_flg/1 -> Switch2/2
  VEPSS_StrWhlTqReqAst_Nm/1 -> MotorTorqueRequestCalculation/1(VEPSS_StrWhlTqReqAst_Nm)
  VEPSS_StrWhlTqReqTq_Nm/1 -> MotorTorqueRequestCalculation/2(VEPSS_StrWhlTqReqTq_Nm)
  VEPSS_StrWhlTqReqAng_Nm/1 -> MotorTorqueRequestCalculation/3(VEPSS_StrWhlTqReqAng_Nm)
  VEPSS_TorqueModeActive_flg/1 -> MotorTorqueRequestCalculation/4(VEPSS_TorqueModeActive_flg)
  VEPSS_AngleModeActive_flg/1 -> MotorTorqueRequestCalculation/5(VEPSS_AngleModeActive_flg)
  VISP_VehSpd_kph/1 -> MotorTorqueRequestCalculation/6(VISP_VehSpd_kph)
  VISP_LFCTransGain_rat/1 -> MotorTorqueRequestCalculation/7(VISP_LFCTransGain_rat)
  VISP_LFCTransGainAppl_flg/1 -> MotorTorqueRequestCalculation/8(VISP_LFCTransGainAppl_flg)
  MotorPWMRequestCalculation/1(VEPSS_EPSMotPWMReqRaw_pct) -> Switch2/1
  VISP_EPSModeReq_enum/1 -> MotorTorqueRequestCalculation/10(VISP_EPSModeReq_enum)

== system hcu_main_ADASwEPS/EPSS/EPSS/EPSTest ==
  PassThrough : Inport
  Amplitude_pct : Constant  Value=5
  Compare To Constant : simulink/Logic and Bit Operations/Compare To Constant  relop===  const=3.0  OutDataTypeStr=boolean
  Constant : Constant  Value=2*pi  OutDataTypeStr=single
  Frequency_Hz : Constant
  Multiport Switch1 : MultiPortSwitch  Inputs=4
  PWMSetPt : Constant
  Product : Product  Inputs=3  RndMeth=Zero
  Product1 : Product  RndMeth=Zero
  SignalPlayer : Subsystem
  TestMode_Sw : Constant
  Timer : Subsystem
  Trigonometric Funcon : Trigonometry
  PWMOut : Outport
  wires:
  Multiport Switch1/1 -> PWMOut/1  "PWMOut"
  PassThrough/1 -> Multiport Switch1/2
  PWMSetPt/1 -> Multiport Switch1/3
  Product1/1 -> Multiport Switch1/4
  Frequency_Hz/1 -> Product/2
  Product/1 -> Trigonometric Funcon/1
  Amplitude_pct/1 -> Product1/2
  Trigonometric Funcon/1 -> Product1/1
  Constant/1 -> Product/3
  Timer/1(SineTime_s) -> Product/1
  TestMode_Sw/1 -> SignalPlayer/1(In1), Compare To Constant/1, Multiport Switch1/1
  Compare To Constant/1 -> Timer/Enable
  SignalPlayer/1(Out1) -> Multiport Switch1/5

== system hcu_main_ADASwEPS/EPSS/EPSS/InternalMode ==
  VEPSS_EPSTqOnShaftFlt_Nm : Inport
  VISP_StrTqReq_Nm : Inport  Port=2
  VISP_StrTqReqAppl_flg : Inport  Port=3
  VISP_EPSModeReq_enum : Inport  Port=4
  VISP_ADASLKAStatus_enum : Inport  Port=5
  VISP_ADASLFCStatus_enum : Inport  Port=6
  Constant1 : Constant  Value=ENUM_LKACCONTSTATUS_ACTIVE
  Constant10 : Constant  Value=ENUM_ADASLKASTATUS_OFF
  Constant11 : Constant  Value=ENUM_LKACCONTSTATUS_NOTAVAIL_TEMP
  Constant2 : Constant  Value=ENUM_ADASLFCSTATUS_OFF
  Constant3 : Constant  Value=ENUM_LKACCONTSTATUS_READY
  Constant5 : Constant  Value=ENUM_LKACCONTSTATUS_ACTIVE
  Constant6 : Constant  Value=ENUM_EPSMODEREQ_INTERNAL
  Constant7 : Constant  Value=ENUM_ADASLKASTATUS_ACTIVE
  Constant8 : Constant  Value=ENUM_LKACCONTSTATUS_OFF
  Constant9 : Constant  Value=ENUM_ADASLKASTATUS_STANDBY
  Logical Operator : Logic  Inputs=4  AllPortsSameDT=off  OutDataTypeStr=boolean
  Relational Operator{1..6} (6 alike) : RelationalOperator  Operator===  OutDataTypeStr=boolean
  Sum : Sum
  Switch{1,4..6} (4 alike) : Switch  Criteria=u2 ~= 0
  VEPSS_StrWhlTqReqAst_Nm : Outport
  VEPSS_LKAContStatus_enum : Outport  Port=2
  wires:
  VEPSS_EPSTqOnShaftFlt_Nm/1 -> Sum/2, Switch4/3
  Constant5/1 -> Relational Operator2/2
  [VEPSS_LKAContStatus_enum] -> Relational Operator2/1
  VISP_StrTqReq_Nm/1 -> Sum/1
  Switch4/1 -> VEPSS_StrWhlTqReqAst_Nm/1  "VEPSS_StrWhlTqReqAst_Nm"
  Switch1/1 -> VEPSS_LKAContStatus_enum/1, [VEPSS_LKAContStatus_enum]  "VEPSS_LKAContStatus_enum"
  Constant1/1 -> Switch1/1
  VISP_EPSModeReq_enum/1 -> Relational Operator3/1
  Constant6/1 -> Relational Operator3/2
  VISP_StrTqReqAppl_flg/1 -> Logical Operator/1
  Logical Operator/1 -> Switch1/2
  Relational Operator3/1 -> Logical Operator/3
  Constant7/1 -> Relational Operator4/2
  Relational Operator4/1 -> Logical Operator/4
  Switch5/1 -> Switch1/3
  Constant9/1 -> Relational Operator5/2
  Relational Operator5/1 -> Switch5/2
  Constant3/1 -> Switch5/1
  Switch6/1 -> Switch5/3
  VISP_ADASLKAStatus_enum/1 -> Relational Operator6/1, Relational Operator5/1, Relational Operator4/1
  Constant10/1 -> Relational Operator6/2
  Relational Operator6/1 -> Switch6/2
  Constant8/1 -> Switch6/1
  Constant11/1 -> Switch6/3
  VISP_ADASLFCStatus_enum/1 -> Relational Operator1/1
  Constant2/1 -> Relational Operator1/2
  Relational Operator1/1 -> Logical Operator/2
  Relational Operator2/1 -> Switch4/2
  Sum/1 -> Switch4/1

== system hcu_main_ADASwEPS/EPSS/EPSS/InverseAssistTable ==
  1/KSTR_PWM2TqGain_rat : Gain  Gain=0.09
  MSTR_EPSMotPWMRescalingInv_pct : Lookup  InputValues=[-250 -3 0 3 250]  Table=[-100 -3 0 3 100]  LookUpMeth=Interpolation-Use End Values
      settings: AttributesFormatString="Input=\"%<InputValues>\"\\nOutput=\"%<Table>\""
  MSTR_TqAssistPWM_pct : Lookup  InputValues=[-20 -19 -18 -17 -16 -15 -14 -13 -12 -11 -10 -9 -8 -7 -6 -5 -4 -3 -2 -1 0 1 2 3 4 5 6 7 8 9 10 11 12 13 14 15 16 17 18 19 20]  Table=[-10:0.5:10]  LookUpMeth=Interpolation-Use End Values
      settings: AttributesFormatString="Input=\"%<InputValues>\"\\nOutput=\"%<Table>\""
  MSTR_VehSpdPWMMult_rat : Lookup  InputValues=[-100 -80 -60 -40 -20 -10 0 10 20 40 60 80 100]  Table=[1 1 1 1 1 1 1 1 1 1 1 1 1]  LookUpMeth=Interpolation-Use End Values
      settings: AttributesFormatString="Input=\"%<InputValues>\"\\nOutput=\"%<Table>\""
  Product : Product  Inputs=*/
  Terminator : Terminator
  VDINR_VehSpd_kph : Constant  Value=0
  VSTR_EPSMotTqReq_Nm : Constant  Value=0
  wires:
  MSTR_EPSMotPWMRescalingInv_pct/1 -> Product/1
  VSTR_EPSMotTqReq_Nm/1 -> 1/KSTR_PWM2TqGain_rat/1
  1/KSTR_PWM2TqGain_rat/1 -> MSTR_EPSMotPWMRescalingInv_pct/1
  VDINR_VehSpd_kph/1 -> MSTR_VehSpdPWMMult_rat/1
  MSTR_VehSpdPWMMult_rat/1 -> Product/2
  Product/1 -> MSTR_TqAssistPWM_pct/1
  MSTR_TqAssistPWM_pct/1 -> Terminator/1  "VSTR_StrWheelTqReq_Nm"

== system hcu_main_ADASwEPS/EPSS/EPSS/LFCStatusArbitration ==
  VISP_EPSModeReq_enum : Inport
  VEPSS_LFCContStatusAng_enum : Inport  Port=2
  VEPSS_LFCContStatusTq_enum : Inport  Port=3
  Constant6 : Constant  Value=ENUM_EPSMODEREQ_ANGLE
  Relational Operator3 : RelationalOperator  Operator===  OutDataTypeStr=boolean
  Switch1 : Switch  Criteria=u2 ~= 0
  VEPSS_LFCContStatus_enum : Outport
  wires:
  VISP_EPSModeReq_enum/1 -> Relational Operator3/1
  Constant6/1 -> Relational Operator3/2
  Relational Operator3/1 -> Switch1/2
  VEPSS_LFCContStatusAng_enum/1 -> Switch1/1
  VEPSS_LFCContStatusTq_enum/1 -> Switch1/3
  Switch1/1 -> VEPSS_LFCContStatus_enum/1

== system hcu_main_ADASwEPS/EPSS/EPSS/PWM Output Limit ==
  VEPSS_SteerPWM_pct : Inport
  VISP_StrAng_deg : Inport  Port=2
  VISP_StrAngValid_flg : Inport  Port=3
  Data Type Conversion : DataTypeConversion
  KEPSS_LockLimitationDefault_rat : Constant  SampleTime=-1
  KEPSS_MotorDutyMaxLim_pct : Constant  Value=100  SampleTime=-1
  KEPSS_MotorDutyMinLim_pct : Constant  Value=-100  SampleTime=-1
  Limit : adas_lib/Limit
  MEPSS_LockLimitation_rat : Lookup  InputValues=[-600 -540 0 540 600]  Table=[0.5 1 1 1 0.5]  LookUpMeth=Interpolation-Use End Values
      settings: AttributesFormatString="Input=\"%<InputValues>\"\\nOutput=\"%<Table>\""
  Product : Product
  Switch : Switch  Criteria=u2 ~= 0
  VEPSS_MotorDuty_pct_over : adas_lib/Signal_over  parent_name=VEPSS_MotorDuty_pct  cal=0
  VEPSS_MotorDuty_pct : Outport
  wires:
  VEPSS_SteerPWM_pct/1 -> Limit/1
  VEPSS_MotorDuty_pct_over/1 -> Data Type Conversion/1
  KEPSS_MotorDutyMaxLim_pct/1 -> Limit/2
  KEPSS_MotorDutyMinLim_pct/1 -> Limit/3
  Data Type Conversion/1 -> VEPSS_MotorDuty_pct/1  "VEPSS_MotorDuty_pct"
  VISP_StrAng_deg/1 -> MEPSS_LockLimitation_rat/1
  MEPSS_LockLimitation_rat/1 -> Switch/1
  VISP_StrAngValid_flg/1 -> Switch/2
  KEPSS_LockLimitationDefault_rat/1 -> Switch/3
  Limit/1 -> Product/1
  Product/1 -> VEPSS_MotorDuty_pct_over/1
  Switch/1 -> Product/2  "VEPSS_LockLimitation_rat"

== system hcu_main_ADASwEPS/EPSS/EPSS/ShaftTorqueProcessor ==
  VISP_EPSTqOnShaft_Nm : Inport
  Data Type Conversion : DataTypeConversion
  NotchFilter1 : DiscreteTransferFcn  Numerator=[1 -1.994058244407765 0.995032825431470]  Denominator=[1 -1.974205875760737 0.975180456784442]
  NotchFilter2 : DiscreteTransferFcn  Numerator=[1 -1.991175781675417 0.993076280925535]  Denominator=[1 -1.963525487771149 0.965425987021267]
  NotchFilter3 : DiscreteTransferFcn  Numerator=[1 -1.986359097364601 0.990196128638903]  Denominator=[1 -1.941183460066831 0.945020491341134]
  NotchFilter4 : DiscreteTransferFcn  Numerator=[1 -1.978872423909787 0.986339393241381]  Denominator=[1 -1.924580367084394 0.932047336415988]
  NotchFilter5 : DiscreteTransferFcn  Numerator=[1 -1.956033818662219 0.973851168649108]  Denominator=[1 -1.853080945250230 0.870898295237120]
  VEPSS_EPSTqOnShaftRaw_Nm : Outport
  VEPSS_EPSTqOnShaftFlt_Nm : Outport  Port=2
  wires:
  VISP_EPSTqOnShaft_Nm/1 -> Data Type Conversion/1, NotchFilter1/1
  NotchFilter1/1 -> NotchFilter2/1
  NotchFilter2/1 -> NotchFilter3/1
  NotchFilter3/1 -> NotchFilter4/1
  NotchFilter4/1 -> NotchFilter5/1
  NotchFilter5/1 -> VEPSS_EPSTqOnShaftFlt_Nm/1  "VEPSS_EPSTqOnShaftFlt_Nm"
  Data Type Conversion/1 -> VEPSS_EPSTqOnShaftRaw_Nm/1  "VEPSS_EPSTqOnShaftRaw_Nm"
